simulink library "eats_dpSimple_generic_std"  (Simulink 8.3)
settings: Solver=ode45  StartTime=0.0  StopTime=10.0  RelTol=1e-3
undefined symbols (not defined in the file): sMP
settings Model: Creator=rafrey5  LastModifiedBy=gerhajo

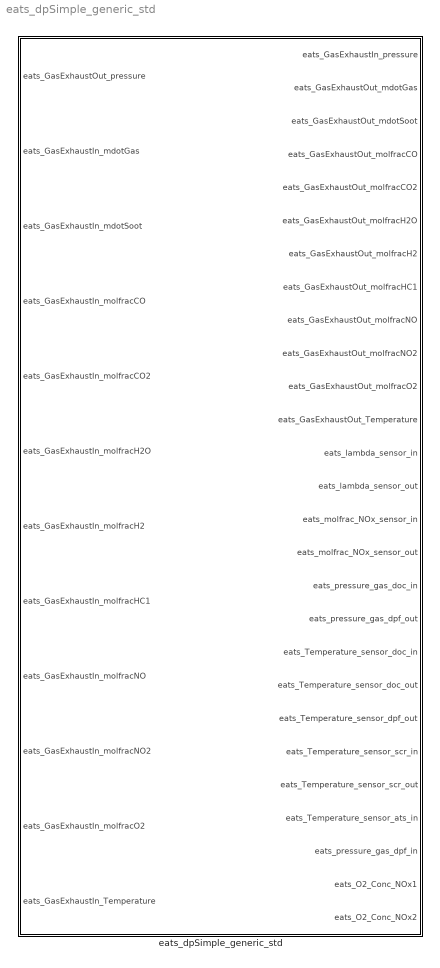
== system eats_dpSimple_generic_std ==
  eats_dpSimple_generic_std : Subsystem  mask(DIVe MB dpSimple){dp_linear=sMP.phys.eats.dp_linear, dp_quadratic=sMP.phys.eats.dp_quadratic, eats_GasExhaustIn_pressure=sMP.phys.eats.out.eats_GasExhaustIn_pressure, eats_GasExhaustOut_mdotGas=sMP.phys.eats.out.eats_GasExhaustOut_mdotGas, eats_GasExhaustOut_mdotSoot=sMP.phys.eats.out.eats_GasExhaustOut_mdotSoot, eats_GasExhaustOut_molfracCO=sMP.phys.eats.out.eats_GasExhaustOut_molfracCO, eats_GasExhaustOut_molfracCO2=sMP.phys.eats.out.eats_GasExhaustOut_molfracCO2, eats_GasExhaustOut_molfracH2O=sMP.phys.eats.out.eats_GasExhaustOut_molfracH2O, eats_GasExhaustOut_molfracHC1=sMP.phys.eats.out.eats_GasExhaustOut_molfracHC1, eats_GasExhaustOut_molfracNO=sMP.phys.eats.out.eats_GasExhaustOut_molfracNO, eats_GasExhaustOut_molfracNO2=sMP.phys.eats.out.eats_GasExhaustOut_molfracNO2, eats_GasExhaustOut_molfracO2=sMP.phys.eats.out.eats_GasExhaustOut_molfracO2, eats_GasExhaustOut_Temperature=sMP.phys.eats.out.eats_GasExhaustOut_Temperature, eats_lambda_sensor_in=sMP.phys.eats.out.eats_lambda_sensor_in, eats_lambda_sensor_out=sMP.phys.eats.out.eats_lambda_sensor_out, eats_molfrac_NOx_sensor_in=sMP.phys.eats.out.eats_molfrac_NOx_sensor_in, eats_molfrac_NOx_sensor_out=sMP.phys.eats.out.eats_molfrac_NOx_sensor_out, eats_pressure_gas_doc_in=sMP.phys.eats.out.eats_pressure_gas_doc_in, eats_pressure_gas_dpf_out=sMP.phys.eats.out.eats_pressure_gas_dpf_out, eats_Temperature_sensor_doc_in=sMP.phys.eats.out.eats_Temperature_sensor_doc_in, eats_Temperature_sensor_doc_out=sMP.phys.eats.out.eats_Temperature_sensor_doc_out, eats_Temperature_sensor_dpf_out=sMP.phys.eats.out.eats_Temperature_sensor_dpf_out, eats_Temperature_sensor_scr_in=sMP.phys.eats.out.eats_Temperature_sensor_scr_in, eats_Temperature_sensor_scr_out=sMP.phys.eats.out.eats_Temperature_sensor_scr_out, SensorGain_NOXRAW=sMP.phys.eats.SensorGain_NOXRAW, SensorOffset_NOXRAW=sMP.phys.eats.SensorOffset_NOXRAW, GasExhaustIn_pressureGain=sMP.phys.eats.GasExhaustIn_pressureGain}
      mask prompts: dp_linear "Pressure drop linear factor [-]:"; dp_quadratic "Pressure drop quadratic factor [-]:"; eats_GasExhaustIn_pressure "Pressure exhaust gas EATS inlet constant [mbar]:"; eats_GasExhaustOut_mdotGas "Massflow exhaust gas EATS outlet constant [kg/s]:"; eats_GasExhaustOut_mdotSoot "Soot massflow exhaust gas EATS outlet constant [g/h]:"; eats_GasExhaustOut_molfracCO "CO molar fraction exhaust gas EATS outlet constant [ppm]:"; eats_GasExhaustOut_molfracCO2 "CO2 molar fraction exhaust gas EATS outlet constant [-]:"; eats_GasExhaustOut_molfracH2O "H2O molar fraction exhaust gas EATS outlet constant [-]:"; eats_GasExhaustOut_molfracHC1 "HC1 molar fraction exhaust gas EATS outlet constant [ppm]:"; eats_GasExhaustOut_molfracNO "NO molar fraction exhaust gas EATS outlet constant [ppm]:"; eats_GasExhaustOut_molfracNO2 "NO2 molar fraction exhaust gas EATS outlet constant [ppm]:"; eats_GasExhaustOut_molfracO2 "O2 molar fraction exhaust gas EATS outlet constant [-]:"; eats_GasExhaustOut_Temperature "Temperature exhaust gas EATS outlet constant [°C]:"; eats_lambda_sensor_in "Lambda exhaust gas EATS inlet constant [-]:"; eats_lambda_sensor_out "Lambda exhaust gas EATS outlet constant [-]:"; eats_molfrac_NOx_sensor_in "NOx molar fraction exhaust gas EATS inlet (sensor) constant [ppm]:"; eats_molfrac_NOx_sensor_out "NOx molar fraction exhaust gas EATS outlet (sensor) constant [ppm]:"; eats_pressure_gas_doc_in "Pressure exhaust gas before DOC constant [mbar]:"; eats_pressure_gas_dpf_out "Pressure exhaust gas after DPF constant [mbar]:"; eats_Temperature_sensor_doc_in "Temperature exhaust gas before DOC (sensor) constant [°C]:"; eats_Temperature_sensor_doc_out "Temperature exhaust gas after DOC (sensor) constant [°C]:"; eats_Temperature_sensor_dpf_out "Temperature exhaust gas after DPF (sensor) constant [°C]:"; eats_Temperature_sensor_scr_in "Temperature exhaust gas before SCR (sensor) constant [°C]:"; eats_Temperature_sensor_scr_out "Temperature exhaust gas after SCR (sensor) constant [°C]:"
      mask help: This block provides an exhaust pressure loss which behaves linear-quadratic on the exhaust volume flow according the MDES test bench converntions for the exhaust flap control at the test bench.
      mask Help: This block provides an exhaust pressure loss which behaves linear-quadratic on the exhaust volume flow according the MDES test bench converntions for the exhaust flap control at the test bench.

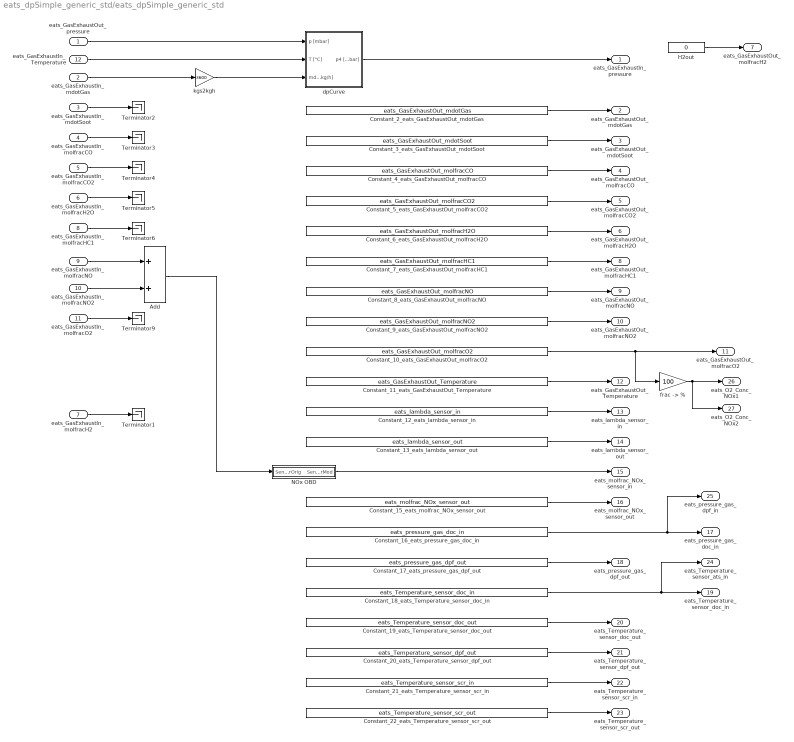
== system eats_dpSimple_generic_std/eats_dpSimple_generic_std ==
  eats_GasExhaustOut_pressure : Inport
  eats_GasExhaustIn_mdotGas : Inport  Port=2
  eats_GasExhaustIn_mdotSoot : Inport  Port=3
  eats_GasExhaustIn_molfracCO : Inport  Port=4
  eats_GasExhaustIn_molfracCO2 : Inport  Port=5
  eats_GasExhaustIn_molfracH2O : Inport  Port=6
  eats_GasExhaustIn_molfracH2 : Inport  Port=7
  eats_GasExhaustIn_molfracHC1 : Inport  Port=8
  eats_GasExhaustIn_molfracNO : Inport  Port=9
  eats_GasExhaustIn_molfracNO2 : Inport  Port=10
  eats_GasExhaustIn_molfracO2 : Inport  Port=11
  eats_GasExhaustIn_Temperature : Inport  Port=12
  Add : Sum
  Constant_10_eats_GasExhaustOut_molfracO2 : Constant  Value=eats_GasExhaustOut_molfracO2
  Constant_11_eats_GasExhaustOut_Temperature : Constant  Value=eats_GasExhaustOut_Temperature
  Constant_12_eats_lambda_sensor_in : Constant  Value=eats_lambda_sensor_in
  Constant_13_eats_lambda_sensor_out : Constant  Value=eats_lambda_sensor_out
  Constant_15_eats_molfrac_NOx_sensor_out : Constant  Value=eats_molfrac_NOx_sensor_out
  Constant_16_eats_pressure_gas_doc_in : Constant  Value=eats_pressure_gas_doc_in
  Constant_17_eats_pressure_gas_dpf_out : Constant  Value=eats_pressure_gas_dpf_out
  Constant_18_eats_Temperature_sensor_doc_in : Constant  Value=eats_Temperature_sensor_doc_in
  Constant_19_eats_Temperature_sensor_doc_out : Constant  Value=eats_Temperature_sensor_doc_out
  Constant_20_eats_Temperature_sensor_dpf_out : Constant  Value=eats_Temperature_sensor_dpf_out
  Constant_21_eats_Temperature_sensor_scr_in : Constant  Value=eats_Temperature_sensor_scr_in
  Constant_22_eats_Temperature_sensor_scr_out : Constant  Value=eats_Temperature_sensor_scr_out
  Constant_2_eats_GasExhaustOut_mdotGas : Constant  Value=eats_GasExhaustOut_mdotGas
  Constant_3_eats_GasExhaustOut_mdotSoot : Constant  Value=eats_GasExhaustOut_mdotSoot
  Constant_4_eats_GasExhaustOut_molfracCO : Constant  Value=eats_GasExhaustOut_molfracCO
  Constant_5_eats_GasExhaustOut_molfracCO2 : Constant  Value=eats_GasExhaustOut_molfracCO2
  Constant_6_eats_GasExhaustOut_molfracH2O : Constant  Value=eats_GasExhaustOut_molfracH2O
  Constant_7_eats_GasExhaustOut_molfracHC1 : Constant  Value=eats_GasExhaustOut_molfracHC1
  Constant_8_eats_GasExhaustOut_molfracNO : Constant  Value=eats_GasExhaustOut_molfracNO
  Constant_9_eats_GasExhaustOut_molfracNO2 : Constant  Value=eats_GasExhaustOut_molfracNO2
  H2out : Constant  Value=0
  NOx OBD : Subsystem  mask{SensorOffset=SensorOffset_NOXRAW, SensorGain=SensorGain_NOXRAW}
      mask prompts: SensorOffset "sensor offset"; SensorGain "sensor gain"
  Terminator{1..6,9} (7 alike) : Terminator
  dpCurve : Subsystem
  "frac -> %" : Gain  Gain=100
  kgs2kgh : Gain  Gain=3600
  eats_GasExhaustIn_pressure : Outport
  eats_GasExhaustOut_mdotGas : Outport  Port=2
  eats_GasExhaustOut_mdotSoot : Outport  Port=3
  eats_GasExhaustOut_molfracCO : Outport  Port=4
  eats_GasExhaustOut_molfracCO2 : Outport  Port=5
  eats_GasExhaustOut_molfracH2O : Outport  Port=6
  eats_GasExhaustOut_molfracH2 : Outport  Port=7
  eats_GasExhaustOut_molfracHC1 : Outport  Port=8
  eats_GasExhaustOut_molfracNO : Outport  Port=9
  eats_GasExhaustOut_molfracNO2 : Outport  Port=10
  eats_GasExhaustOut_molfracO2 : Outport  Port=11
  eats_GasExhaustOut_Temperature : Outport  Port=12
  eats_lambda_sensor_in : Outport  Port=13
  eats_lambda_sensor_out : Outport  Port=14
  eats_molfrac_NOx_sensor_in : Outport  Port=15
  eats_molfrac_NOx_sensor_out : Outport  Port=16
  eats_pressure_gas_doc_in : Outport  Port=17
  eats_pressure_gas_dpf_out : Outport  Port=18
  eats_Temperature_sensor_doc_in : Outport  Port=19
  eats_Temperature_sensor_doc_out : Outport  Port=20
  eats_Temperature_sensor_dpf_out : Outport  Port=21
  eats_Temperature_sensor_scr_in : Outport  Port=22
  eats_Temperature_sensor_scr_out : Outport  Port=23
  eats_Temperature_sensor_ats_in : Outport  Port=24
  eats_pressure_gas_dpf_in : Outport  Port=25
  eats_O2_Conc_NOx1 : Outport  Port=26
  eats_O2_Conc_NOx2 : Outport  Port=27
  wires:
  eats_GasExhaustIn_mdotSoot/1 -> Terminator2/1
  eats_GasExhaustIn_molfracCO/1 -> Terminator3/1
  eats_GasExhaustIn_molfracCO2/1 -> Terminator4/1
  eats_GasExhaustIn_molfracH2O/1 -> Terminator5/1
  eats_GasExhaustIn_molfracHC1/1 -> Terminator6/1
  eats_GasExhaustIn_molfracNO/1 -> Add/1
  eats_GasExhaustIn_molfracNO2/1 -> Add/2
  eats_GasExhaustIn_molfracO2/1 -> Terminator9/1
  Constant_2_eats_GasExhaustOut_mdotGas/1 -> eats_GasExhaustOut_mdotGas/1
  Constant_3_eats_GasExhaustOut_mdotSoot/1 -> eats_GasExhaustOut_mdotSoot/1
  Constant_4_eats_GasExhaustOut_molfracCO/1 -> eats_GasExhaustOut_molfracCO/1
  Constant_5_eats_GasExhaustOut_molfracCO2/1 -> eats_GasExhaustOut_molfracCO2/1
  Constant_6_eats_GasExhaustOut_molfracH2O/1 -> eats_GasExhaustOut_molfracH2O/1
  Constant_7_eats_GasExhaustOut_molfracHC1/1 -> eats_GasExhaustOut_molfracHC1/1
  Constant_8_eats_GasExhaustOut_molfracNO/1 -> eats_GasExhaustOut_molfracNO/1
  Constant_9_eats_GasExhaustOut_molfracNO2/1 -> eats_GasExhaustOut_molfracNO2/1
  Constant_11_eats_GasExhaustOut_Temperature/1 -> eats_GasExhaustOut_Temperature/1
  Constant_12_eats_lambda_sensor_in/1 -> eats_lambda_sensor_in/1
  Constant_13_eats_lambda_sensor_out/1 -> eats_lambda_sensor_out/1
  Constant_15_eats_molfrac_NOx_sensor_out/1 -> eats_molfrac_NOx_sensor_out/1
  Constant_16_eats_pressure_gas_doc_in/1 -> eats_pressure_gas_dpf_in/1, eats_pressure_gas_doc_in/1
  Constant_17_eats_pressure_gas_dpf_out/1 -> eats_pressure_gas_dpf_out/1
  Constant_18_eats_Temperature_sensor_doc_in/1 -> eats_Temperature_sensor_ats_in/1, eats_Temperature_sensor_doc_in/1
  Constant_19_eats_Temperature_sensor_doc_out/1 -> eats_Temperature_sensor_doc_out/1
  Constant_20_eats_Temperature_sensor_dpf_out/1 -> eats_Temperature_sensor_dpf_out/1
  Constant_21_eats_Temperature_sensor_scr_in/1 -> eats_Temperature_sensor_scr_in/1
  Constant_22_eats_Temperature_sensor_scr_out/1 -> eats_Temperature_sensor_scr_out/1
  eats_GasExhaustOut_pressure/1 -> dpCurve/1(p [mbar])
  eats_GasExhaustIn_Temperature/1 -> dpCurve/2(T [°C])
  eats_GasExhaustIn_mdotGas/1 -> kgs2kgh/1
  kgs2kgh/1 -> dpCurve/3(mdot [kg/h])
  Add/1 -> NOx OBD/1(SensorOrig)
  NOx OBD/1(SensorMod) -> eats_molfrac_NOx_sensor_in/1
  dpCurve/1(p4 [mbar]) -> eats_GasExhaustIn_pressure/1
  Constant_10_eats_GasExhaustOut_molfracO2/1 -> "frac -> %"/1, eats_GasExhaustOut_molfracO2/1
  "frac -> %"/1 -> eats_O2_Conc_NOx2/1, eats_O2_Conc_NOx1/1
  eats_GasExhaustIn_molfracH2/1 -> Terminator1/1
  H2out/1 -> eats_GasExhaustOut_molfracH2/1

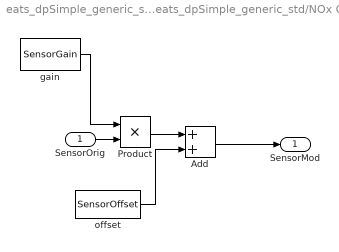
== system eats_dpSimple_generic_std/eats_dpSimple_generic_std/NOx OBD ==
  SensorOrig : Inport
  Add : Sum
  Product : Product  RndMeth=Zero
  gain : Constant  Value=SensorGain
  offset : Constant  Value=SensorOffset
  SensorMod : Outport
  wires:
  gain/1 -> Product/1
  Product/1 -> Add/1
  offset/1 -> Add/2
  SensorOrig/1 -> Product/2
  Add/1 -> SensorMod/1

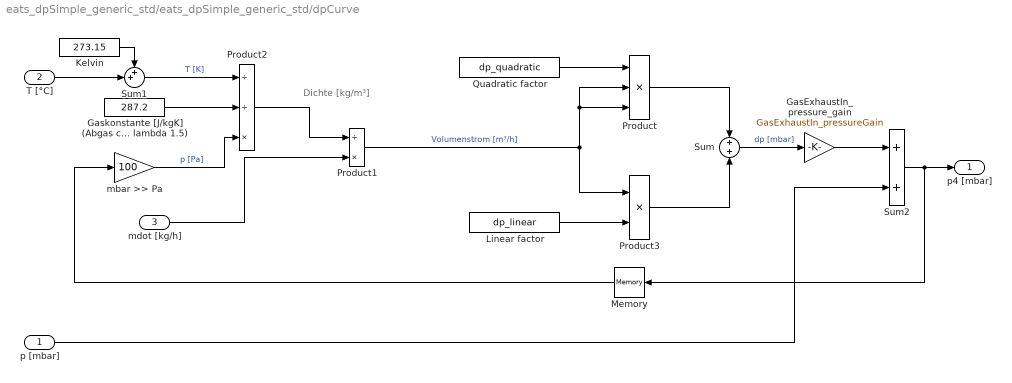
== system eats_dpSimple_generic_std/eats_dpSimple_generic_std/dpCurve ==
  note: Dichte [kg/m³]
  p [mbar] : Inport
  T [°C] : Inport  Port=2
  mdot [kg/h] : Inport  Port=3
  GasExhaustIn_pressure_gain : Gain  Gain=GasExhaustIn_pressureGain
  "Gaskonstante [J/kgK] (Abgas ca 200°C, lambda 1.5)" : Constant  Value=287.2
  Kelvin : Constant  Value=273.15
  Linear factor : Constant  Value=dp_linear
  Memory : Memory  X0=eats_GasExhaustIn_pressure
  Product : Product  Inputs=3  RndMeth=Zero
  Product1 : Product  Inputs=/*  SaturateOnIntegerOverflow=on  InputSameDT=on  OutDataTypeStr=Inherit: Same as first input
  Product2 : Product  Inputs=//*  SaturateOnIntegerOverflow=on  InputSameDT=on  OutDataTypeStr=Inherit: Same as first input
  Product3 : Product  RndMeth=Zero
  Quadratic factor : Constant  Value=dp_quadratic
  Sum : Sum
  Sum1 : Sum  Inputs=++|
  Sum2 : Sum
  mbar >> Pa : Gain  Gain=100
  p4 [mbar] : Outport
  wires:
  Kelvin/1 -> Sum1/1
  T [°C]/1 -> Sum1/2
  Sum1/1 -> Product2/1  "T [K]"
  mbar >> Pa/1 -> Product2/3  "p [Pa]"
  Linear factor/1 -> Product3/2
  Product3/1 -> Sum/2
  Product/1 -> Sum/1
  Quadratic factor/1 -> Product/1
  Product1/1 -> Product3/1, Product/3, Product/2  "Volumenstrom [m³/h]"
  Product2/1 -> Product1/1
  mdot [kg/h]/1 -> Product1/2
  "Gaskonstante [J/kgK] (Abgas ca 200°C, lambda 1.5)"/1 -> Product2/2
  p [mbar]/1 -> Sum2/2
  Sum/1 -> GasExhaustIn_pressure_gain/1  "dp [mbar]"
  Sum2/1 -> p4 [mbar]/1, Memory/1
  Memory/1 -> mbar >> Pa/1
  GasExhaustIn_pressure_gain/1 -> Sum2/1
